simulink model "CD2_WWTP_CD2RUMBA_v01"  (Simulink 6.4)
settings: Solver=FixedStepDiscrete  StartTime=0  StopTime=12000  FixedStep=300  RelTol=1e-3
undefined symbols (not defined in the file or in its folder): CD2_get_substances_count
settings Model: LastModifiedBy=c81523
settings DataIOCC: LimitDataPoints=off  TimeSaveName=cd_time  SignalLoggingName=sigsOut
settings DebuggingCC: SolverPrmCheckMsg=none  StrictBusMsg=None
settings HardwareCC: TargetUnknown=on

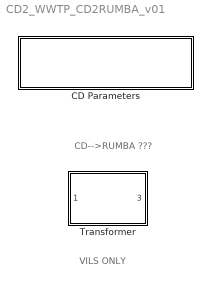
== system CD2_WWTP_CD2RUMBA_v01 ==
  note: CD-->RUMBA ???
  note: VILS ONLY
  CD Parameters : Subsystem  mask(City Drain 1.0 - Simulation parameters ){t_step=300, t_start=0, t_stop=12000}
      mask prompts: t_step "Sampling Time [s]"; t_start "Start Time [s]"; t_stop "Stop Time [s]"
      mask help:
      | Block that sets the global parameters required in City Drain 1.0. Following paramters are set without user's input:
      |
      | - 'Solver' --> 'FixedStepDiscrete'
      | - 'TimeSaveName' --> 'cd_time'
      | - 'Decimation' --> '1'
      | - 'LimitDataPoints' -->  'off'
      mask init:
      | % toplevel systems' name --> Plant file name;
      | tls=bdroot(gcb); 
      | set_param(tls, 'Solver', 'FixedStepDiscrete'); 
      | set_param(tls, 'TimeSaveName', 'cd_time');
      | set_param(tls, 'Decimation', '1');
      | set_param(tls, 'LimitDataPoints', 'off');
      | set_param(tls, 'ScreenColor', 'white');
      | 
      | tstep_char=num2str(t_step); % Setting the discrete time step
      | set_param(tls, 'FixedStep', tstep_char); 
      | 
      | tstart_char=num2str(t_start); % Setting the start time
      | set_param(tls, 'StartTime', tstart_char); 
      | 
      | tstop_char=num2str(t_stop); % Setting the stop time
      | set_param(tls, 'StopTime', tstop_char);
      mask Display:
      | plot(0,0,100,100);
      | 
      | text(50,65,'CITY DRAIN','HorizontalAlignment','center');
      | text(50,35,'PARAMETERS','HorizontalAlignment','center');
      | 
      | 
      | image(imread('CityDrain_SimParam.jpg'))
  Transformer : Subsystem  mask(WWTP Trans){n_comp=CD2_get_substances_count}
      mask prompts: n_comp "Number of pollutants [ - ]"
      mask help:
      | Function used:
      | CD2_sfun_trans.m
      mask init:
      | % reading the toplevel systems' name 
      | % --> Plant file name;
      | tls=bdroot(gcb); 
      | % Obtaining the fixed sampling time
      | t_samp_char=get_param(tls, 'FixedStep');
      | % Convertion to numeric value
      | tstep = str2num(t_samp_char);
      mask Display:
      | plot(0,0,100,100);
      | 
      | 
      | text(50,60,'WWTP','HorizontalAlignment','center');
      | text(50,40,'Trans','HorizontalAlignment','center');
      | 
      | 
      | port_label('input',1,'Qi');
      | port_label('output',1,'S');

== system CD2_WWTP_CD2RUMBA_v01/CD Parameters ==

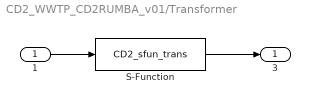
== system CD2_WWTP_CD2RUMBA_v01/Transformer ==
  " 1" : Inport
  S-Function : S-Function  FunctionName=CD2_sfun_trans  Parameters=n_comp,tstep
  " 3" : Outport
  wires:
  " 1"/1 -> S-Function/1
  S-Function/1 -> " 3"/1
